simulink model "Eg5_16"  (R2018a)
settings: Solver=VariableStepAuto  StartTime=0.0  StopTime=10.0  RelTol=1e-3
libraries: simulink x1
settings Model: Creator=wangluo  LastModifiedBy=wangluo

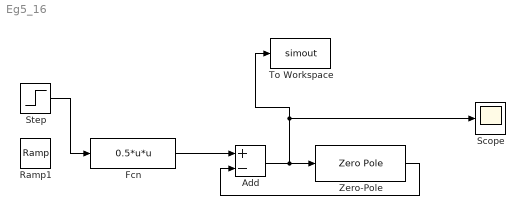
== system Eg5_16 ==
  Add : Sum  Inputs=+-
  Fcn : Fcn  Expr=0.5*u*u
  Ramp1 : simulink/Sources/Ramp  slope=1  start=0  InitialOutput=0
  Scope : Scope
  Step : Step  SampleTime=0
  To Workspace : ToWorkspace  VariableName=simout  SaveFormat=Timeseries  SampleTime=-1
  Zero-Pole : ZeroPole  Zeros=[-5]  Poles=[0 0 -10]
  wires:
  Fcn/1 -> Add/1
  Add/1 -> To Workspace/1, Scope/1, Zero-Pole/1
  Zero-Pole/1 -> Add/2
  Step/1 -> Fcn/1
